simulink model "LC_teszt"  (R2019b)
settings: Solver=VariableStepAuto  StartTime=0.0  StopTime=0.5  RelTol=1e-3
undefined symbols (not defined in the file): C_dhs, L_dhs
settings Model: Creator=kissd  LastModifiedBy=kissd

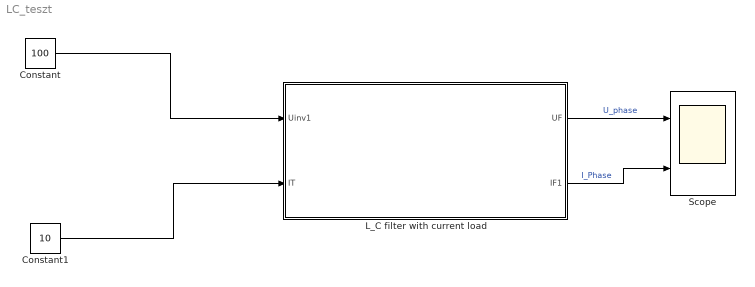
== system LC_teszt ==
  Constant : Constant  Value=100
  Constant1 : Constant  Value=10
  L_C filter with current load : Subsystem
  Scope : Scope  NumInputPorts=2
  wires:
  Constant/1 -> L_C filter with current load/1(Uinv1)
  L_C filter with current load/1(UF) -> Scope/1  "U_phase"
  L_C filter with current load/2(IF1) -> Scope/2  "I_Phase"
  Constant1/1 -> L_C filter with current load/2(IT)

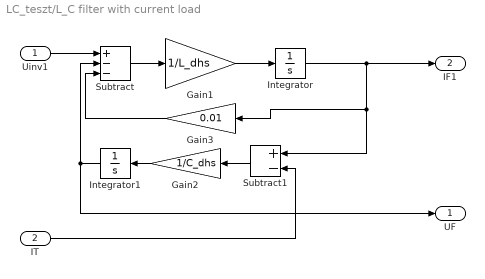
== system LC_teszt/L_C filter with current load ==
  Uinv1 : Inport
  IT : Inport  Port=2
  Gain1 : Gain  Gain=1/L_dhs
  Gain2 : Gain  Gain=1/C_dhs
  Gain3 : Gain  Gain=0.01
  Integrator : Integrator
  Integrator1 : Integrator
  Subtract : Sum  Inputs=+--
  Subtract1 : Sum  Inputs=+-
  UF : Outport
  IF1 : Outport  Port=2
  wires:
  Integrator1/1 -> UF/1, Subtract/2
  Subtract/1 -> Gain1/1
  Gain1/1 -> Integrator/1
  Integrator/1 -> Gain3/1, Subtract1/1, IF1/1
  IT/1 -> Subtract1/2
  Gain2/1 -> Integrator1/1
  Uinv1/1 -> Subtract/1
  Subtract1/1 -> Gain2/1
  Gain3/1 -> Subtract/3
